simulink model "VFcontrolFINAL"  (R2013b)
settings: Solver=ode45  StartTime=0.0  StopTime=5  RelTol=1e-3
libraries: powerlib x20, powerlib_meascontrol x4
settings Model: Creator=Somesh  LastModifiedBy=Somesh
settings DataIOCC: SignalLoggingSaveFormat=ModelDataLogs
settings OptimizationCC: ExpressionDepthLimit=2147483647
settings DebuggingCC: FcnCallInpInsideContextMsg=EnableAllAsWarning  StateNameClashWarn=warning
settings GRTTargetCC: CombineOutputUpdateFcns=off  GRTInterface=on

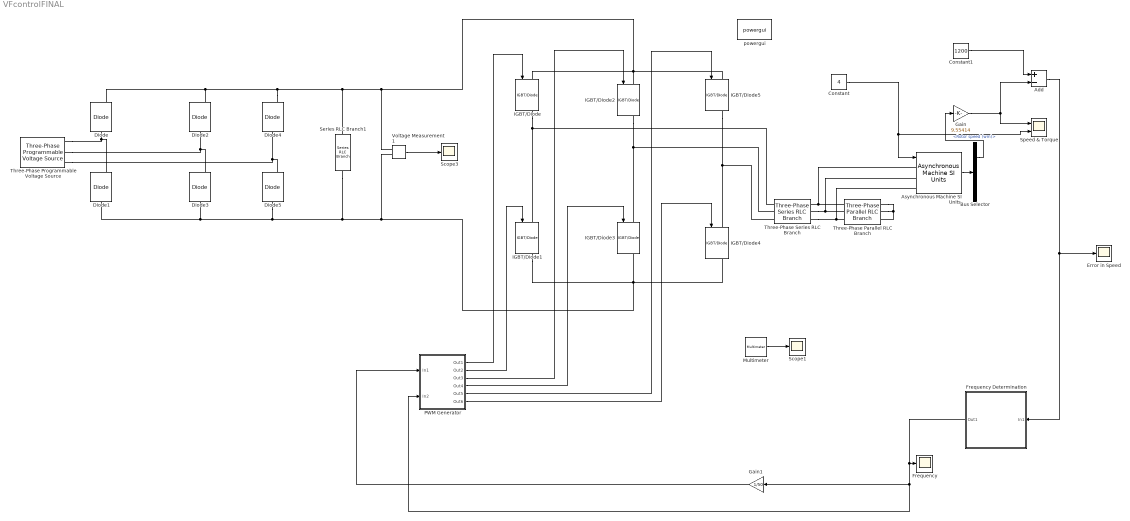
== system VFcontrolFINAL ==
  Add : Sum  Inputs=+-
  Asynchronous Machine SI Units : powerlib/Machines/Asynchronous Machine SI Units  PresetModel="15:  5.4 HP (4KW)   400 V  50Hz 1430 RPM"  MechanicalLoad=Torque Tm  ShowDetailedParameters=on  RotorType=Squirrel-cage  ReferenceFrame=Stationary  NominalParameters=[4000 400 50]  Stator=[1.405 0.005839]  Rotor=[1.395 0.005839]  Cage1=[ 0.022 0.226/377]  Cage2=[ 0.022 0.226/377]  Lm=0.1722  Mechanical=[0.0131 0.002985 2]  PolePairs=2  InitialConditions=[1 0 0 0 0 0 0 0]  Units=SI  LoadFlowParameters=1492000  SimulateSaturation=off  Saturation=[14.03593122, 27.81365428, 53.79336849, 72.68890987, 97.98006896, 148.6815601, 215.7428561, 302.9841135, 428.7778367 ; 230, 322, 414, 460, 506, 552, 598, 644, 690]  TsPowergui=0  TsBlock=-1  IterativeModel=Forward Euler  Pmec=0
  Bus Selector : BusSelector  OutputSignals=Mechanical.Rotor speed (wm),Mechanical.Electromagnetic torque Te (N*m)
  Constant : Constant  Value=4
  Constant1 : Constant  Value=1200
  Diode{,1..5} (6 alike) : powerlib/Power Electronics/Diode  Ron=0.001  Lon=0  Vf=0.8  IC=0  UseSnubber=off  Rs=500  Cs=250e-9  Measurements=on
  Error in Speed : Scope
      settings: YMin=0.765  YMax=0.84  SaveName=ScopeData4
  Frequency : Scope
      settings: YMin=38.57  YMax=42.63  SaveName=ScopeData2
  Frequency Determination : Subsystem
  Gain : Gain  Gain=9.55414
  Gain1 : Gain  Gain=1/50
  IGBT/Diode{,1..5} (6 alike) : powerlib/Power Electronics/IGBT//Diode  Ron=1e-3  Rs=1e5  Cs=inf  Measurements=on
  Multimeter : powerlib/Measurements/Multimeter  PhasorSimulation=off  OutputType=Complex  sel=[1 2 3]  L=3  Gain=[1 1 1]  yselected={'Ub1: Three-Phase Parallel RLC Branch','Ub2: Three-Phase Parallel RLC Branch','Ub3: Three-Phase Parallel RLC Branch'};  PSBOutputType=1  PSBequivalent=0  AxesSetting=[0,0.1,-100,100]  Display=1  SavedBlockNames=-11
  PWM Generator : Subsystem
  Scope1 : Scope
      settings: YMin=-250  YMax=250
  Scope3 : Scope
      settings: YMin=472.43  YMax=472.62  SaveName=ScopeData6
  Series RLC Branch1 : powerlib/Elements/Series RLC Branch  LConnTagsString=__new0  RConnTagsString=__new0  BranchType=C  Resistance=1  Inductance=1e-3  SetiL0=off  InitialCurrent=0  Capacitance=1  Setx0=off  InitialVoltage=0  Measurements=None
  Speed & Torque : Scope  NumInputPorts=2
      settings: YMin=1200.43~3.8  YMax=1200.49~4.2  SaveName=ScopeData3
  Three-Phase Parallel RLC Branch : powerlib/Elements/Three-Phase Parallel RLC Branch  LConnTagsString=A|B|C  RConnTagsString=A|B|C  BranchType=RC  Resistance=20  Inductance=1e-3  Capacitance=1  Measurements=Branch voltages
  Three-Phase Programmable Voltage Source : powerlib/Electrical Sources/Three-Phase Programmable Voltage Source  PositiveSequence="[280  0 50]"  VariationEntity=Amplitude  VariationType=Table of time-amplitude pairs  VariationTypeAlt=Step  VariationStep=0.5  VariationRate=10  VariationMagnitude=0.3  VariationFrequency=2  VariationTiming=[1 2]  VariationPhaseA=off  Amplitudes=[1 0.8 1.2 1.0]  TimeValues=[0 0.1 0.15 0.2]  HarmonicGeneration=off  HarmonicA=[3 0.2 -25 0]  HarmonicB=[2 0.15 35 2]  Timing="[0.05  3]"  BusType=swing  Pref=0  Qref=0  Qmin=-inf  Qmax=inf
  Three-Phase Series RLC Branch : powerlib/Elements/Three-Phase Series RLC Branch  LConnTagsString=A|B|C  RConnTagsString=A|B|C  BranchType=L  Resistance=1  Inductance=1e-5  Capacitance=1e-6  Measurements=None
  Voltage Measurement1 : powerlib/Measurements/Voltage Measurement  PhasorSimulation=off  OutputType=Complex  PSBequivalent=0
  powergui : powerlib/powergui  Priority=1  SimulationMode=Continuous  SolverType=Tustin  SampleTime=50e-6  frequency=60  SPID=off  DisableSnubberDevices=off  DisableRonSwitches=off  DisableVfSwitches=off  SwTol=0  Interpol=off  DisplayEquations=off  frequencyindice=0  Pbase=100e6  ErrMax=1e-4  Iterations=50  UnitsV=kV  UnitsW=MW  FunctionMessages=off  echomessages=off  HookPort=off  EnableUseOfTLC=off  x0status=blocks  RestoreLinks=warning  ResistiveCurrentMeasurement=off  Frange=[0:2:500]  Ylog=off  Xlog=on  ShowGrid=off  save=off  variable=ZData  ZoomFFT=off  StartTime=0.0  cycles=1  DisplayStyle=1  fundamental=60  FreqAxis=off  MaxFrequency=1000  frequencyindicesteady=1  RmsSteady=1  display=off  Ts=0  methode=off
  wires:
  PWM Generator/1(Out1) -> IGBT/Diode/1
  PWM Generator/3(Out3) -> IGBT/Diode2/1
  PWM Generator/5(Out5) -> IGBT/Diode5/1
  PWM Generator/2(Out2) -> IGBT/Diode1/1
  PWM Generator/4(Out4) -> IGBT/Diode3/1
  PWM Generator/6(Out6) -> IGBT/Diode4/1
  Multimeter/1 -> Scope1/1
  Asynchronous Machine SI Units/1 -> Bus Selector/1
  Bus Selector/1 -> Gain/1  "<Rotor speed (wm)>"
  Gain/1 -> Speed & Torque/1, Add/2
  Constant1/1 -> Add/1
  Add/1 -> Error in Speed/1, Frequency Determination/1(In1)
  Frequency Determination/1(Out1) -> PWM Generator/2(In2), Gain1/1, Frequency/1
  Constant/1 -> Asynchronous Machine SI Units/1, Speed & Torque/2
  Gain1/1 -> PWM Generator/1(In1)
  Voltage Measurement1/1 -> Scope3/1
  connections:
  IGBT/Diode5/RConn1 -- Three-Phase Series RLC Branch/LConn3 -- IGBT/Diode4/LConn1
  Diode4/RConn1 -- Series RLC Branch1/LConn1 -- Voltage Measurement1/LConn1 -- IGBT/Diode5/LConn1 -- IGBT/Diode2/LConn1 -- IGBT/Diode/LConn1 -- Diode/RConn1 -- Diode2/RConn1
  IGBT/Diode2/RConn1 -- Three-Phase Series RLC Branch/LConn2 -- IGBT/Diode3/LConn1
  IGBT/Diode/RConn1 -- Three-Phase Series RLC Branch/LConn1 -- IGBT/Diode1/LConn1
  Diode5/LConn1 -- Series RLC Branch1/RConn1 -- IGBT/Diode1/RConn1 -- IGBT/Diode3/RConn1 -- IGBT/Diode4/RConn1 -- Voltage Measurement1/LConn2 -- Diode1/LConn1 -- Diode3/LConn1
  Diode/LConn1 -- Three-Phase Programmable Voltage Source/RConn1 -- Diode1/RConn1
  Diode2/LConn1 -- Three-Phase Programmable Voltage Source/RConn2 -- Diode3/RConn1
  Diode4/LConn1 -- Three-Phase Programmable Voltage Source/RConn3 -- Diode5/RConn1
  Three-Phase Parallel RLC Branch/RConn3 -- Three-Phase Parallel RLC Branch/RConn2 -- Three-Phase Parallel RLC Branch/RConn1
  Three-Phase Parallel RLC Branch/LConn3 -- Asynchronous Machine SI Units/LConn3 -- Three-Phase Series RLC Branch/RConn3
  Three-Phase Parallel RLC Branch/LConn2 -- Asynchronous Machine SI Units/LConn2 -- Three-Phase Series RLC Branch/RConn2
  Three-Phase Parallel RLC Branch/LConn1 -- Asynchronous Machine SI Units/LConn1 -- Three-Phase Series RLC Branch/RConn1

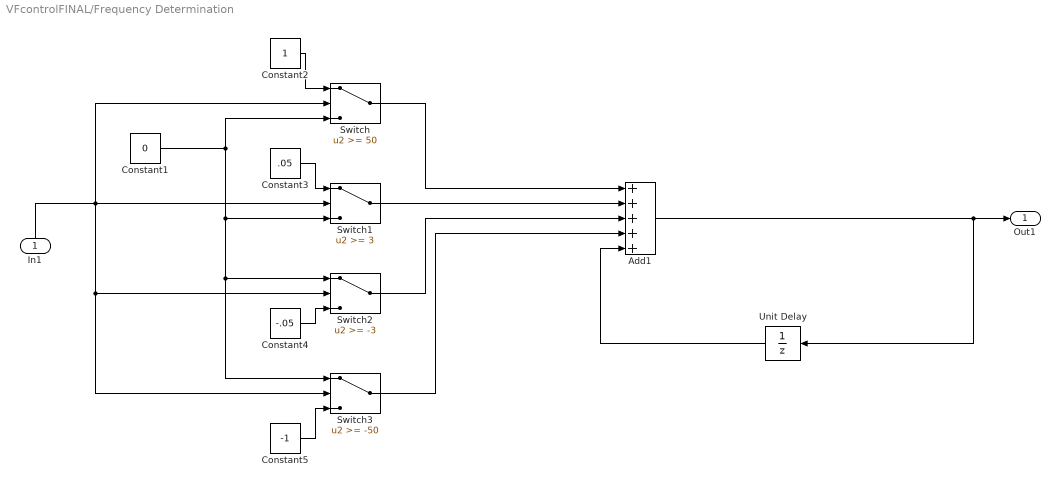
== system VFcontrolFINAL/Frequency Determination ==
  In1 : Inport
  Add1 : Sum  Inputs=+++++  SampleTime=.02
  Constant1 : Constant  Value=0
  Constant2 : Constant
  Constant3 : Constant  Value=.05
  Constant4 : Constant  Value=-.05
  Constant5 : Constant  Value=-1
  Switch : Switch  Threshold=50
  Switch1 : Switch  Threshold=3
  Switch2 : Switch  Threshold=-3
  Switch3 : Switch  Threshold=-50
  Unit Delay : UnitDelay  InitialCondition=50  SampleTime=.02
  Out1 : Outport
  wires:
  Constant2/1 -> Switch/1
  Constant1/1 -> Switch/3, Switch1/3, Switch2/1, Switch3/1
  Constant3/1 -> Switch1/1
  Constant4/1 -> Switch2/3
  Constant5/1 -> Switch3/3
  Switch/1 -> Add1/1
  Switch1/1 -> Add1/2
  Switch2/1 -> Add1/3
  Switch3/1 -> Add1/4
  Unit Delay/1 -> Add1/5
  In1/1 -> Switch/2, Switch1/2, Switch2/2, Switch3/2
  Add1/1 -> Unit Delay/1, Out1/1

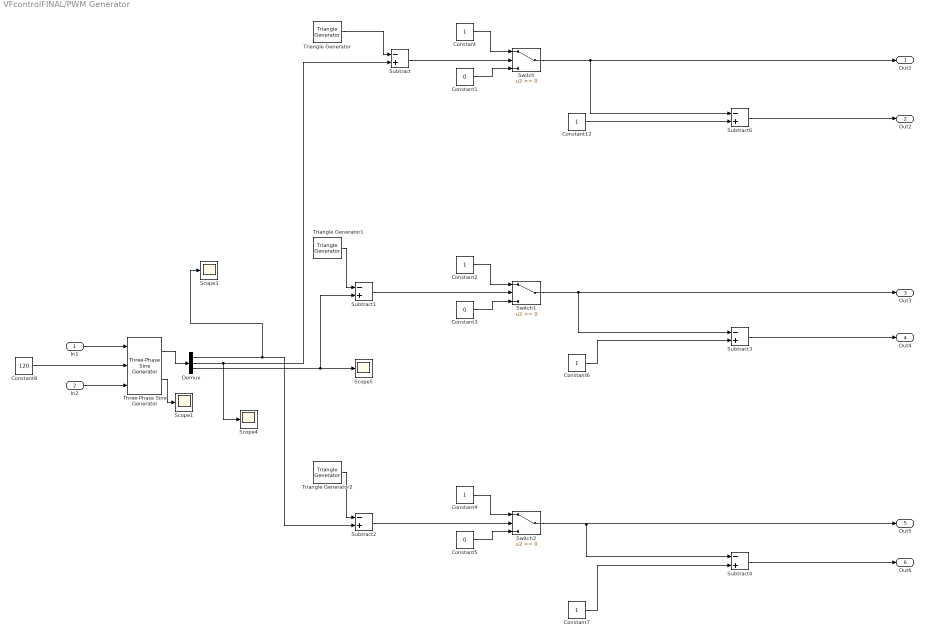
== system VFcontrolFINAL/PWM Generator ==
  In1 : Inport
  In2 : Inport  Port=2
  Constant{,2,4,6..7,12} (6 alike) : Constant
  Constant1 : Constant  Value=0
  Constant3 : Constant  Value=0
  Constant5 : Constant  Value=0
  Constant8 : Constant  Value=120
  Demux : Demux  Outputs=3
  Scope{1,3..5} (4 alike) : Scope
      Scope1 settings: YMin=-250  YMax=250
      Scope3 settings: YMin=-250  YMax=250
      Scope4 settings: YMin=-250  YMax=250  SaveName=ScopeData2
      Scope5 settings: YMin=-250  YMax=250  SaveName=ScopeData3
  Subtract{,1..4,6} (6 alike) : Sum  Inputs=-+
  Switch : Switch
  Switch1 : Switch
  Switch2 : Switch
  Three-Phase Sine Generator : powerlib_meascontrol/Pulse & Signal Generators/Three-Phase Sine Generator  Ts=0
  Triangle Generator : powerlib_meascontrol/Pulse & Signal Generators/Triangle Generator  Freq=31*50  Phase=0  Ts=0
  Triangle Generator1 : powerlib_meascontrol/Pulse & Signal Generators/Triangle Generator  Freq=31*50  Phase=0  Ts=0
  Triangle Generator2 : powerlib_meascontrol/Pulse & Signal Generators/Triangle Generator  Freq=31*50  Phase=0  Ts=0
  Out1 : Outport
  Out2 : Outport  Port=2
  Out3 : Outport  Port=3
  Out4 : Outport  Port=4
  Out5 : Outport  Port=5
  Out6 : Outport  Port=6
  wires:
  Triangle Generator/1 -> Subtract/1
  Demux/2 -> Subtract/2, Scope4/1
  Subtract/1 -> Switch/2
  Constant1/1 -> Switch/3
  Constant/1 -> Switch/1
  Switch/1 -> Out1/1, Subtract6/1
  Constant12/1 -> Subtract6/2
  Subtract6/1 -> Out2/1
  Triangle Generator1/1 -> Subtract1/1
  Subtract1/1 -> Switch1/2
  Constant3/1 -> Switch1/3
  Constant2/1 -> Switch1/1
  Triangle Generator2/1 -> Subtract2/1
  Subtract2/1 -> Switch2/2
  Constant5/1 -> Switch2/3
  Constant4/1 -> Switch2/1
  Switch1/1 -> Out3/1, Subtract3/1
  Constant6/1 -> Subtract3/2
  Constant7/1 -> Subtract4/2
  Switch2/1 -> Out5/1, Subtract4/1
  Subtract4/1 -> Out6/1
  Subtract3/1 -> Out4/1
  In1/1 -> Three-Phase Sine Generator/1
  Constant8/1 -> Three-Phase Sine Generator/2
  In2/1 -> Three-Phase Sine Generator/3
  Three-Phase Sine Generator/1 -> Demux/1
  Demux/1 -> Scope3/1, Subtract2/2
  Demux/3 -> Scope5/1, Subtract1/2
  Three-Phase Sine Generator/2 -> Scope1/1
